simulink model "PI_controller_alpha0"  (R2019b)
settings: Solver=FixedStepAuto  StartTime=0.0  StopTime=5  FixedStep=0.005  RelTol=1e-3
settings Model: Creator=suvo  LastModifiedBy=suvo

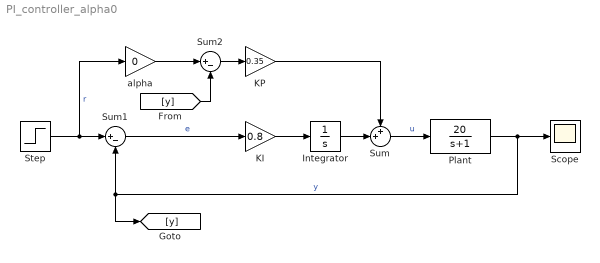
== system PI_controller_alpha0 ==
  Integrator : Integrator
  KI : Gain  Gain=0.8
  KP : Gain  Gain=0.35
  Plant : TransferFcn  Numerator=20  Denominator=[1 1]
  Scope : Scope
  Step : Step  SampleTime=0
  Sum : Sum  Inputs=++|
  Sum1 : Sum  Inputs=|+-
  Sum2 : Sum  Inputs=|+-
  alpha : Gain  Gain=0
  wires:
  KI/1 -> Integrator/1
  Sum1/1 -> KI/1  "e"
  Plant/1 -> Scope/1, [y], Sum1/2  "y"
  Step/1 -> alpha/1, Sum1/1  "r"
  Sum2/1 -> KP/1
  KP/1 -> Sum/1
  Integrator/1 -> Sum/2
  Sum/1 -> Plant/1  "u"
  [y] -> Sum2/2
  alpha/1 -> Sum2/1
